simulink model "MRACArduino"  (R2022a)
settings: Solver=FixedStepAuto  StartTime=0.0  StopTime=inf  RelTol=1e-3  EnableMultiTasking=on
undefined symbols (not defined in the file): a_m, b_m, c
libraries: arduinolib x2
settings Model: ExtModeTrigDuration=2  Creator=edgar  LastModifiedBy=edgar
settings OptimizationCC: EnhancedBackFolding=on  PassReuseOutputArgsAs=Individual arguments  ZeroExternalMemoryAtStartup=off  ZeroInternalMemoryAtStartup=off  MaxStackSize=64  OptimizeBlockOrder=speed  DifferentSizesBufferReuse=on  OptimizationCustomize=off  EfficientTunableParamExpr=on
settings DebuggingCC: ParameterTunabilityLossMsg=error
settings HardwareCC: ProdBitPerInt=16  ProdBitPerPointer=16  ProdBitPerSizeT=16  ProdBitPerPtrDiffT=16  ProdLargestAtomicFloat=None  ProdWordSize=8  ProdHWDeviceType=Atmel->AVR
settings SFSimCC: MATLABDynamicMemAlloc=off
settings RTWCC: SystemTargetFile=ert.tlc  HardwareBoard=Arduino Uno  TemplateMakefile=ert_default_tmf  Toolchain=Arduino AVR  BuildConfiguration=Faster Runs
settings CodeAppCC: ForceParamTrailComments=on  IgnoreCustomStorageClasses=off  OperatorAnnotations=on  SimulinkDataObjDesc=on  SFDataObjDesc=on  InsertBlockDesc=on
settings ERTTargetCC: SupportContinuousTime=on  SupportVariableSizeSignals=on  ExtModeTransport=3  ExtModeStaticAlloc=on  ExtModeStaticAllocSize=250  ExtModeMexFile=ext_xcp  ExtModeIntrfLevel=Level2 - Open

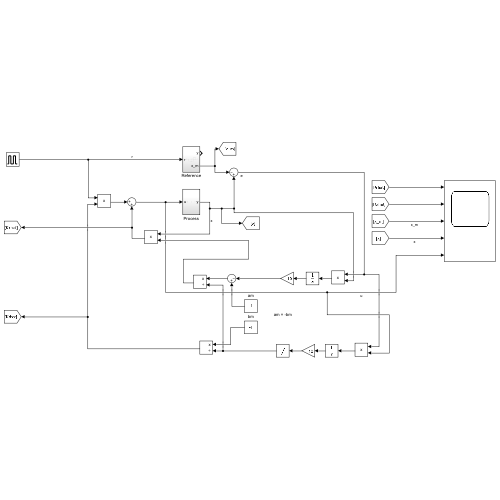
[thumbnail: Simulink's stored preview of the top-level diagram]
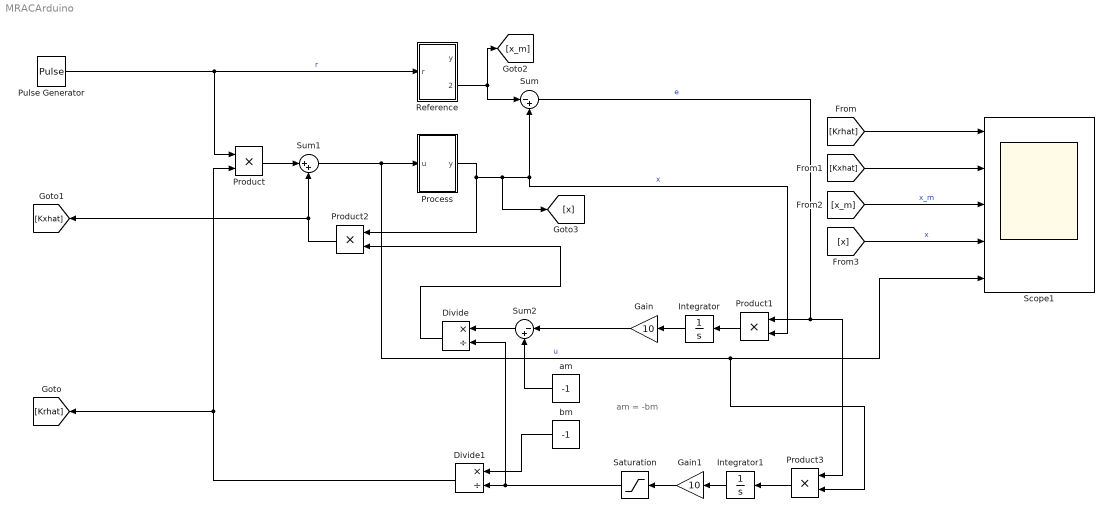
== system MRACArduino ==
  note: am = -bm
  Divide : Product  Inputs=*/
  Divide1 : Product  Inputs=*/
  Gain : Gain  Gain=10
  Gain1 : Gain  Gain=10
  Integrator : Integrator  InitialCondition=1
  Integrator1 : Integrator  InitialCondition=1
  Process : Subsystem
  Product{,1..3} (4 alike) : Product
  Pulse Generator : DiscretePulseGenerator  PulseType=Time based  Period=5  PulseWidth=50
  Reference : Subsystem
  Saturation : Saturate  UpperLimit=1000  LowerLimit=0.1
  Scope1 : Scope  NumInputPorts=5
  Sum : Sum  Inputs=|-+
  Sum1 : Sum  Inputs=|++
  Sum2 : Sum  Inputs=|-+
  am : Constant  Value=-1
  bm : Constant  Value=-1
  wires:
  am/1 -> Sum2/2
  Divide1/1 -> [Krhat], Product/2
  [Kxhat] -> Scope1/2
  Pulse Generator/1 -> Product/1, Reference/1(r)  "r"
  Integrator/1 -> Gain/1
  [x_m] -> Scope1/3  "x_m"
  Reference/2(x_m) -> [x_m], Sum/1
  Product2/1 -> [Kxhat], Sum1/2
  Process/1(y) -> Product2/1, Product1/2, Sum/2, [x]  "x"
  Integrator1/1 -> Gain1/1
  [x] -> Scope1/4  "x"
  Product/1 -> Sum1/1
  Divide/1 -> Product2/2
  [Krhat] -> Scope1/1
  Saturation/1 -> Divide/2, Divide1/2
  Product1/1 -> Integrator/1
  Sum1/1 -> Scope1/5, Product3/2, Process/1(u)  "u"
  Sum2/1 -> Divide/1
  Gain1/1 -> Saturation/1
  bm/1 -> Divide1/1
  Gain/1 -> Sum2/1
  Product3/1 -> Integrator1/1
  Sum/1 -> Product1/1, Product3/1  "e"

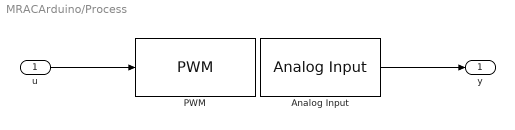
== system MRACArduino/Process ==
  u : Inport
  Analog Input : arduinolib/Analog Input  pinNumber=4  ReadResultsOnly=off  ConversionTriggerSource=Software  ExternalTriggerType=uint32( 0 )  OutputDataType=uint16  EnableConversionCompleteNotify=off  EnableOuputStatus=off  SampleTime=-1  blockPlatform=arduino
  PWM : arduinolib/PWM  pinNumber=5  frequencyType=Default  desiredFrequency=490.2  achievableFrequency=490.2
  y : Outport
  wires:
  u/1 -> PWM/1
  Analog Input/1 -> y/1

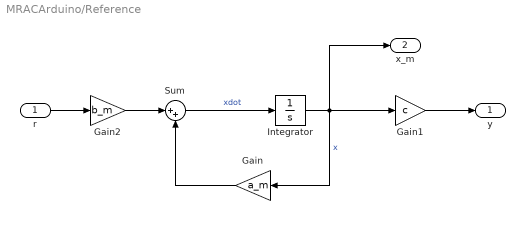
== system MRACArduino/Reference ==
  r : Inport
  Gain : Gain  Gain=a_m
  Gain1 : Gain  Gain=c
  Gain2 : Gain  Gain=b_m
  Integrator : Integrator
  Sum : Sum  Inputs=|++
  y : Outport
  x_m : Outport  Port=2
  wires:
  Sum/1 -> Integrator/1  "xdot"
  Integrator/1 -> x_m/1, Gain1/1, Gain/1  "x"
  Gain1/1 -> y/1
  Gain2/1 -> Sum/1
  Gain/1 -> Sum/2
  r/1 -> Gain2/1
